simulink model "funkcia3"  (R2020a)
settings: Solver=VariableStepAuto  StartTime=0.0  StopTime=40  RelTol=1e-6
libraries: simulink x1
settings Model: Creator=Gani  LastModifiedBy=xacha
settings DataIOCC: ReturnWorkspaceOutputs=off
settings DebuggingCC: ArithmeticOperatorsInVariantConditions=warning
settings SFSimCC: SimUseLocalCustomCode=off  CustomCodeUndefinedFunction=UseInterfaceOnly
settings RTWCC: RTWUseLocalCustomCode=off

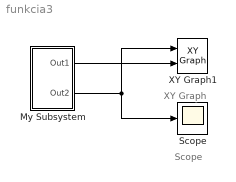
== system funkcia3 ==
  note: Scope
  note: XY Graph
  My Subsystem : Subsystem  mask{a=1, b=1}
      mask prompts: a "input a"; b "input b"
      mask DialogControl DescGroupVar Prompt: Subsystem For All Values
      mask DialogControl DescTextVar Prompt: y"-a*y'-b*y=cos(a*x-1)
      mask DialogControl ParameterGroupVar Prompt: Input Your Values
  Scope : Scope
  XY Graph1 : simulink/Sinks/XY Graph  xmin=-0.5  xmax=0.8  ymin=-2  ymax=2  st=-1
  wires:
  My Subsystem/2(Out2) -> Scope/1, XY Graph1/1
  My Subsystem/1(Out1) -> XY Graph1/2

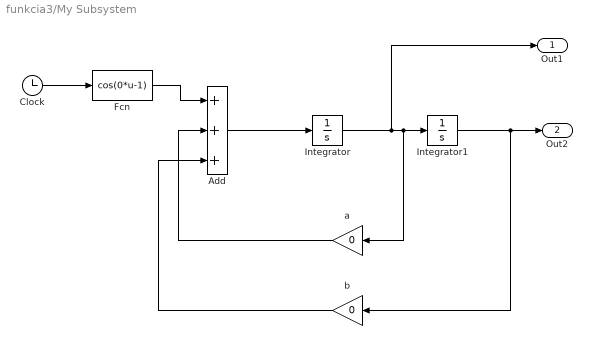
== system funkcia3/My Subsystem ==
  Add : Sum  Inputs=+++
  Clock : Clock
  Fcn : Fcn  Expr=cos(0*u-1)
  Integrator : Integrator
  Integrator1 : Integrator
  a : Gain  Gain=0
  b : Gain  Gain=0
  Out1 : Outport  VectorParamsAs1DForOutWhenUnconnected=off
  Out2 : Outport  Port=2  VectorParamsAs1DForOutWhenUnconnected=off
  wires:
  a/1 -> Add/2
  Fcn/1 -> Add/1
  Integrator1/1 -> Out2/1, b/1
  Integrator/1 -> Out1/1, a/1, Integrator1/1
  Add/1 -> Integrator/1
  b/1 -> Add/3
  Clock/1 -> Fcn/1
